simulink library "eop_grc"  (R2024a)
settings: Solver=VariableStepAuto  StartTime=0.0  StopTime=10.0  RelTol=1e-3
undefined symbols (not defined in the file or in its folder): AEOP_nReqMotSpdMax_X_A, AEOP_nRrOilTempSpdMod_X_degC, AEOP_nRrOilTempSpdMod_Y_KW, AEOP_nRrTMTempSpdMod_X_degC, EopC_bMotEnaMan_C, EopC_bMotEnaManTrig_C, EopC_nReqMotSpdMan_C, EopC_nReqMotSpdMin_C, EopC_nReqMotSpdTrig_C, EopC_rSpdRampDown_C, EopC_rSpdRampUp_C, EopC_volfDmd_A, MEOP_nReqMotSpdMax_Y_T, MEOP_nRrOilTempDetOptMod_Y_T, MEOP_nRrOilTempDetOptMod_Z_M, MEOP_nRrOilTempMotOptMod_Z_M, MEOP_nRrOilTempSpdMod_Z_M, MEOP_nRrTMTempMotOptMod_Y_T, MEOP_nRrTMTempSpdMod_Y_T
libraries: simulink x2
settings Model: Creator=FVT22063  LastModifiedBy=FVT22063

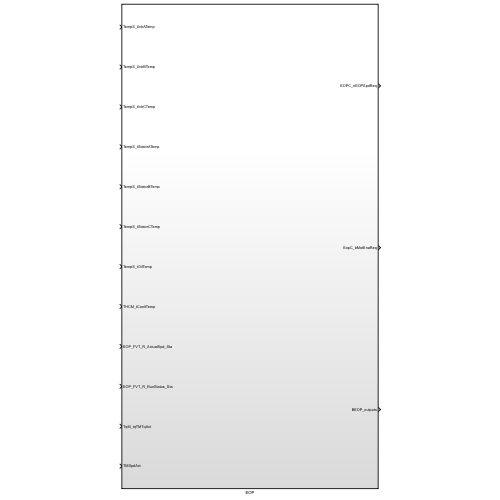
[thumbnail: Simulink's stored preview of the top-level diagram]
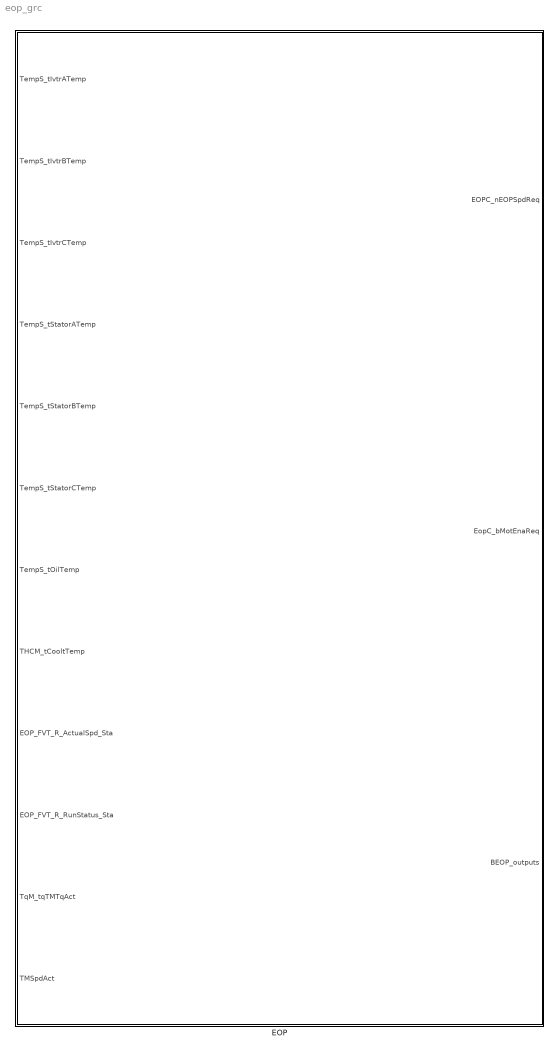
== system eop_grc ==
  EOP : Subsystem  TreatAsAtomicUnit=on
      settings: RTWSystemCode=Nonreusable function  RTWFcnNameOpts=Use subsystem name  RTWFileNameOpts=Use subsystem name

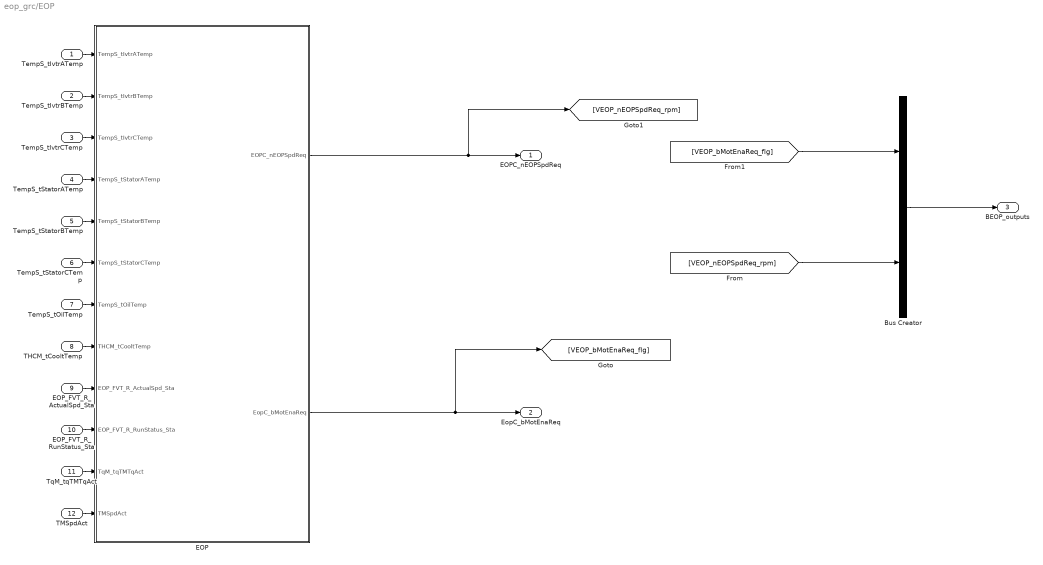
== system eop_grc/EOP ==
  TempS_tIvtrATemp : Inport
  TempS_tIvtrBTemp : Inport  Port=2
  TempS_tIvtrCTemp : Inport  Port=3
  TempS_tStatorATemp : Inport  Port=4
  TempS_tStatorBTemp : Inport  Port=5
  TempS_tStatorCTemp : Inport  Port=6
  TempS_tOilTemp : Inport  Port=7
  THCM_tCooltTemp : Inport  Port=8
  EOP_FVT_R_ActualSpd_Sta : Inport  Port=9
  EOP_FVT_R_RunStatus_Sta : Inport  Port=10
  TqM_tqTMTqAct : Inport  Port=11
  TMSpdAct : Inport  Port=12
  Bus Creator : BusCreator  Inputs=2  OutDataTypeStr=Bus: BEOP_outputs  NonVirtualBus=on
  EOP : Subsystem  TreatAsAtomicUnit=on
  EOPC_nEOPSpdReq : Outport
  EopC_bMotEnaReq : Outport  Port=2
  BEOP_outputs : Outport  Port=3  OutDataTypeStr=Bus: BEOP_outputs
  wires:
  TempS_tStatorBTemp/1 -> EOP/5(TempS_tStatorBTemp)
  TMSpdAct/1 -> EOP/12(TMSpdAct)
  EOP/2(EopC_bMotEnaReq) -> [VEOP_bMotEnaReq_flg], EopC_bMotEnaReq/1
  TempS_tStatorATemp/1 -> EOP/4(TempS_tStatorATemp)
  EOP_FVT_R_RunStatus_Sta/1 -> EOP/10(EOP_FVT_R_RunStatus_Sta)
  EOP_FVT_R_ActualSpd_Sta/1 -> EOP/9(EOP_FVT_R_ActualSpd_Sta)
  TqM_tqTMTqAct/1 -> EOP/11(TqM_tqTMTqAct)
  EOP/1(EOPC_nEOPSpdReq) -> [VEOP_nEOPSpdReq_rpm], EOPC_nEOPSpdReq/1
  TempS_tIvtrBTemp/1 -> EOP/2(TempS_tIvtrBTemp)
  THCM_tCooltTemp/1 -> EOP/8(THCM_tCooltTemp)
  TempS_tIvtrATemp/1 -> EOP/1(TempS_tIvtrATemp)
  TempS_tStatorCTemp/1 -> EOP/6(TempS_tStatorCTemp)
  TempS_tIvtrCTemp/1 -> EOP/3(TempS_tIvtrCTemp)
  TempS_tOilTemp/1 -> EOP/7(TempS_tOilTemp)
  Bus Creator/1 -> BEOP_outputs/1
  [VEOP_bMotEnaReq_flg] -> Bus Creator/1
  [VEOP_nEOPSpdReq_rpm] -> Bus Creator/2

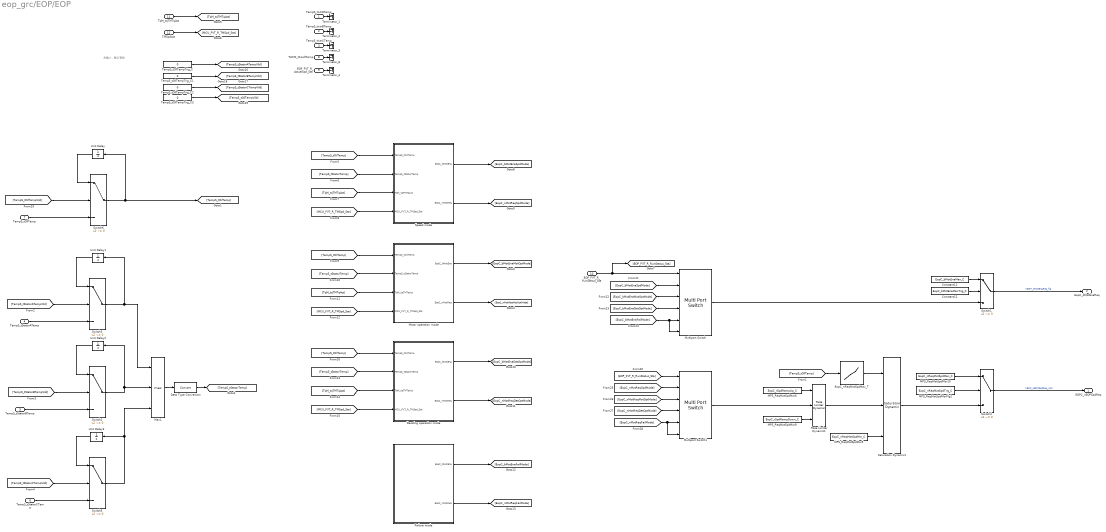
== system eop_grc/EOP/EOP ==
  note: 未输入，默认有效
  TempS_tIvtrATemp : Inport
  TempS_tIvtrBTemp : Inport  Port=2
  TempS_tIvtrCTemp : Inport  Port=3
  TempS_tStatorATemp : Inport  Port=4
  TempS_tStatorBTemp : Inport  Port=5
  TempS_tStatorCTemp : Inport  Port=6
  TempS_tOilTemp : Inport  Port=7
  THCM_tCooltTemp : Inport  Port=8
  EOP_FVT_R_ActualSpd_Sta : Inport  Port=9
  EOP_FVT_R_RunStatus_Sta : Inport  Port=10
  TqM_tqTMTqAct : Inport  Port=11
  TMSpdAct : Inport  Port=12
  Constant11 : Constant  Value=EopC_bMotEnaMan_C
  Constant12 : Constant  Value=EopC_bMotEnaManTrig_C
  Data Type Conversion : DataTypeConversion  SaturateOnIntegerOverflow=off  RndMeth=Floor
  Derating operation mode : Subsystem
  EopC_nReqMotSpdMax_T : Lookup_n-D  NumberOfTableDimensions=1  BreakpointsForDimension1=AEOP_nReqMotSpdMax_X_A  BreakpointsForDimension2=EopC_volfDmd_A  Table=MEOP_nReqMotSpdMax_Y_T  ExtrapMethod=Clip  UseLastTableValue=on  InternalRulePriority=Speed  RndMeth=Simplest
  Failure mode : Subsystem
  MPS_ReqMotSpdMor10 : Constant  Value=EopC_nReqMotSpdMan_C
  MPS_ReqMotSpdMor5 : Constant  Value=EopC_nReqMotSpdMin_C
  MPS_ReqMotSpdMor6 : Constant  Value=EopC_rSpdRampUp_C
  MPS_ReqMotSpdMor9 : Constant  Value=EopC_rSpdRampDown_C
  MPS_ReqMotSpdMorFlg1 : Constant  Value=EopC_nReqMotSpdTrig_C
  Max1 : MinMax  Function=max  Inputs=3
  Motor operation mode : Subsystem
  Multiport Switch : MultiPortSwitch  DataPortOrder=Specify indices  DataPortIndices={0,1,2,3}  DataPortForDefault=Additional data port  DiagnosticForDefault=None  SaturateOnIntegerOverflow=off  InputSameDT=off
  Multiport Switch1 : MultiPortSwitch  DataPortOrder=Zero-based contiguous  Inputs=4  DataPortIndices={EopStsCool.SpdMod, EopStsCool.MotOptMod,EopStsCool.DetOptMod,EopStsCool.FalMod}  DataPortForDefault=Additional data port  DiagnosticForDefault=None  zeroidx=on  SaturateOnIntegerOverflow=off  InputSameDT=off
  Rate Limiter Dynamic1 : simulink/Discontinuities/Rate Limiter Dynamic
  Saturation Dynamic1 : simulink/Discontinuities/Saturation Dynamic  OutMin=[]  OutMax=[]  OutDataTypeStr=Inherit: Same as second input  OutDataType=fixdt(1, 16)  OutScaling=2^-10  DoSatur=off
  Speed mode : Subsystem
  Switch{1..6} (6 alike) : Switch  Criteria=u2 ~= 0  SaturateOnIntegerOverflow=off  InputSameDT=off
  TempS_tOilTempTrig_C{,1..3} (4 alike) : Constant  Value=0
  Terminator_{1..4,8} (5 alike) : Terminator
  Unit Delay{,1..3} (4 alike) : UnitDelay  SampleTime=-1  HasFrameUpgradeWarning=on
  EOPC_nEOPSpdReq : Outport  VectorParamsAs1DForOutWhenUnconnected=off
  EopC_bMotEnaReq : Outport  Port=2  VectorParamsAs1DForOutWhenUnconnected=off
  wires:
  TempS_tIvtrATemp/1 -> Terminator_1/1
  TempS_tIvtrBTemp/1 -> Terminator_2/1
  TempS_tIvtrCTemp/1 -> Terminator_3/1
  TempS_tStatorATemp/1 -> Switch3/3
  THCM_tCooltTemp/1 -> Terminator_8/1
  Switch4/1 -> EOPC_nEOPSpdReq/1  "VEOP_nEOPSpdReq_rpm"
  MPS_ReqMotSpdMor9/1 -> Rate Limiter Dynamic1/3
  Speed mode/2(EopC_nMotReq) -> [EopC_nMotReqSpdMode]
  [EopC_nMotReqDetOptMode] -> Multiport Switch1/4
  [EopC_nMotReqSpdMode] -> Multiport Switch1/2
  [TempS_tOilTemp] -> EopC_nReqMotSpdMax_T/1
  [EopC_bMotEnaMotOptMode] -> Multiport Switch/3
  Speed mode/1(EopC_bMotEna) -> [EopC_bMotEnaSpdMode]
  [EopC_bMotEnaSpdMode] -> Multiport Switch/2
  EOP_FVT_R_RunStatus_Sta/1 -> Multiport Switch/1, [EOP_FVT_R_RunStatus_Sta]
  [EopC_nMotReqFailMode] -> Multiport Switch1/6, Multiport Switch1/5
  MPS_ReqMotSpdMorFlg1/1 -> Switch4/2
  Multiport Switch1/1 -> Rate Limiter Dynamic1/2
  TMSpdAct/1 -> [MCU_FVT_R_TMSpd_Sta]
  Constant12/1 -> Switch1/2
  MPS_ReqMotSpdMor5/1 -> Saturation Dynamic1/3
  [EopC_bMotEnaFailMode] -> Multiport Switch/6, Multiport Switch/5
  Saturation Dynamic1/1 -> Switch4/3
  [EopC_bMotEnaDetOptMode] -> Multiport Switch/4
  EopC_nReqMotSpdMax_T/1 -> Saturation Dynamic1/1
  Multiport Switch/1 -> Switch1/3
  Constant11/1 -> Switch1/1
  [EOP_FVT_R_RunStatus_Sta] -> Multiport Switch1/1
  Switch1/1 -> EopC_bMotEnaReq/1  "VEOP_bMotEnaReq_flg"
  MPS_ReqMotSpdMor10/1 -> Switch4/1
  MPS_ReqMotSpdMor6/1 -> Rate Limiter Dynamic1/1
  [EopC_nMotReqMotOptMode] -> Multiport Switch1/3
  TqM_tqTMTqAct/1 -> [TqM_tqTMTqAct]
  Rate Limiter Dynamic1/1 -> Saturation Dynamic1/2
  TempS_tOilTempTrig_C/1 -> [TempS_tStatorATempVild]
  TempS_tOilTempTrig_C1/1 -> [TempS_tStatorBTempVild]
  TempS_tOilTempTrig_C2/1 -> [TempS_tStatorCTempVild]
  TempS_tOilTempTrig_C3/1 -> [TempS_tOilTempVild]
  Switch3/1 -> Max1/1, Unit Delay1/1
  Unit Delay1/1 -> Switch3/1
  [TempS_tStatorATempVild] -> Switch3/2
  Unit Delay2/1 -> Switch2/1
  Switch2/1 -> Unit Delay2/1, Max1/2
  [TempS_tStatorBTempVild] -> Switch2/2
  TempS_tStatorBTemp/1 -> Switch2/3
  Switch5/1 -> Max1/3, Unit Delay3/1
  Unit Delay3/1 -> Switch5/1
  [TempS_tStatorCTempVild] -> Switch5/2
  TempS_tStatorCTemp/1 -> Switch5/3
  Unit Delay/1 -> Switch6/1
  Switch6/1 -> Unit Delay/1, [TempS_tOilTemp]
  [TempS_tOilTempVild] -> Switch6/2
  TempS_tOilTemp/1 -> Switch6/3
  [TempS_tOilTemp] -> Speed mode/1(TempS_tOilTemp)
  [TempS_tStatorTemp] -> Speed mode/2(TempS_tStatorTemp)
  [MCU_FVT_R_TMSpd_Sta] -> Speed mode/4(MCU_FVT_R_TMSpd_Sta)
  [TqM_tqTMTqAct] -> Speed mode/3(TqM_tqTMTqAct)
  [TqM_tqTMTqAct] -> Motor operation mode/3(TqM_tqTMTqAct)
  [MCU_FVT_R_TMSpd_Sta] -> Motor operation mode/4(MCU_FVT_R_TMSpd_Sta)
  [TempS_tStatorTemp] -> Motor operation mode/2(TempS_tStatorTemp)
  [TempS_tOilTemp] -> Motor operation mode/1(TempS_tOilTemp)
  Motor operation mode/1(EopC_bMotEna) -> [EopC_bMotEnaMotOptMode]
  Motor operation mode/2(EopC_nMotReq) -> [EopC_nMotReqMotOptMode]
  Derating operation mode/2(EopC_nMotReq) -> [EopC_nMotReqDetOptMode]
  Derating operation mode/1(EopC_bMotEna) -> [EopC_bMotEnaDetOptMode]
  [TempS_tOilTemp] -> Derating operation mode/1(TempS_tOilTemp)
  [TempS_tStatorTemp] -> Derating operation mode/2(TempS_tStatorTemp)
  [MCU_FVT_R_TMSpd_Sta] -> Derating operation mode/4(MCU_FVT_R_TMSpd_Sta)
  [TqM_tqTMTqAct] -> Derating operation mode/3(TqM_tqTMTqAct)
  Failure mode/1(EopC_bMotEna) -> [EopC_bMotEnaFailMode]
  Failure mode/2(EopC_nMotReq) -> [EopC_nMotReqFailMode]
  EOP_FVT_R_ActualSpd_Sta/1 -> Terminator_4/1
  Max1/1 -> Data Type Conversion/1
  Data Type Conversion/1 -> [TempS_tStatorTemp]

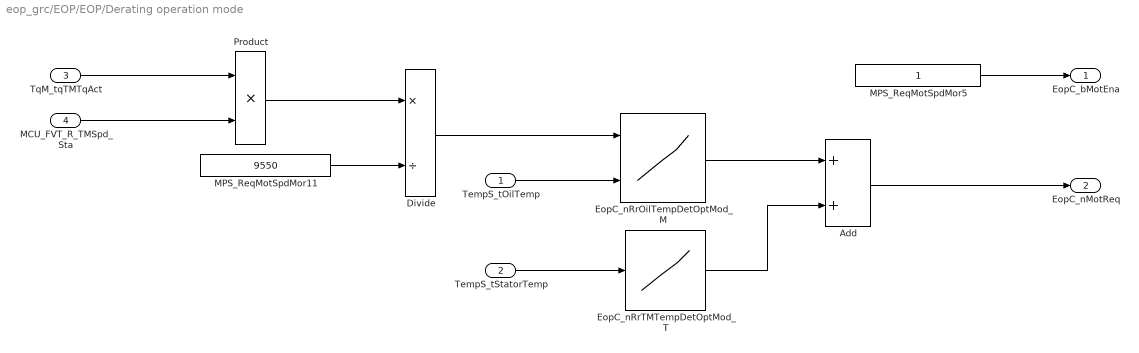
== system eop_grc/EOP/EOP/Derating operation mode ==
  TempS_tOilTemp : Inport
  TempS_tStatorTemp : Inport  Port=2
  TqM_tqTMTqAct : Inport  Port=3
  MCU_FVT_R_TMSpd_Sta : Inport  Port=4
  Add : Sum
  Divide : Product  Inputs=*/
  EopC_nRrOilTempDetOptMod_M : Lookup_n-D  BreakpointsForDimension1=AEOP_nRrOilTempSpdMod_Y_KW  BreakpointsForDimension2=AEOP_nRrOilTempSpdMod_X_degC  Table=MEOP_nRrOilTempDetOptMod_Z_M  ExtrapMethod=Clip  UseLastTableValue=on  InternalRulePriority=Speed  RndMeth=Simplest
      settings: InputPortMap=u0,u1
  EopC_nRrTMTempDetOptMod_T : Lookup_n-D  NumberOfTableDimensions=1  BreakpointsForDimension1=AEOP_nRrTMTempSpdMod_X_degC  BreakpointsForDimension2=EopC_volfDmd_A  Table=MEOP_nRrOilTempDetOptMod_Y_T  ExtrapMethod=Clip  UseLastTableValue=on  InternalRulePriority=Speed  RndMeth=Simplest
  MPS_ReqMotSpdMor11 : Constant  Value=9550  OutDataTypeStr=single
  MPS_ReqMotSpdMor5 : Constant  OutDataTypeStr=boolean
  Product : Product
  EopC_bMotEna : Outport  VectorParamsAs1DForOutWhenUnconnected=off
  EopC_nMotReq : Outport  Port=2  VectorParamsAs1DForOutWhenUnconnected=off
  wires:
  EopC_nRrTMTempDetOptMod_T/1 -> Add/2
  Divide/1 -> EopC_nRrOilTempDetOptMod_M/1
  EopC_nRrOilTempDetOptMod_M/1 -> Add/1
  MPS_ReqMotSpdMor5/1 -> EopC_bMotEna/1
  MPS_ReqMotSpdMor11/1 -> Divide/2
  Product/1 -> Divide/1
  Add/1 -> EopC_nMotReq/1
  TqM_tqTMTqAct/1 -> Product/1
  MCU_FVT_R_TMSpd_Sta/1 -> Product/2
  TempS_tStatorTemp/1 -> EopC_nRrTMTempDetOptMod_T/1
  TempS_tOilTemp/1 -> EopC_nRrOilTempDetOptMod_M/2

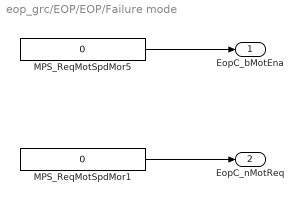
== system eop_grc/EOP/EOP/Failure mode ==
  MPS_ReqMotSpdMor1 : Constant  Value=0  OutDataTypeStr=single
  MPS_ReqMotSpdMor5 : Constant  Value=0  OutDataTypeStr=boolean
  EopC_bMotEna : Outport  VectorParamsAs1DForOutWhenUnconnected=off
  EopC_nMotReq : Outport  Port=2  VectorParamsAs1DForOutWhenUnconnected=off
  wires:
  MPS_ReqMotSpdMor1/1 -> EopC_nMotReq/1
  MPS_ReqMotSpdMor5/1 -> EopC_bMotEna/1

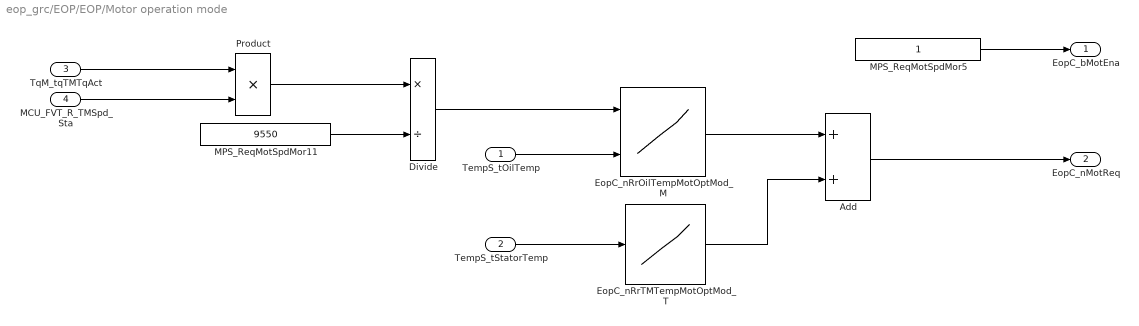
== system eop_grc/EOP/EOP/Motor operation mode ==
  TempS_tOilTemp : Inport
  TempS_tStatorTemp : Inport  Port=2
  TqM_tqTMTqAct : Inport  Port=3
  MCU_FVT_R_TMSpd_Sta : Inport  Port=4
  Add : Sum
  Divide : Product  Inputs=*/
  EopC_nRrOilTempMotOptMod_M : Lookup_n-D  BreakpointsForDimension1=AEOP_nRrOilTempSpdMod_Y_KW  BreakpointsForDimension2=AEOP_nRrOilTempSpdMod_X_degC  Table=MEOP_nRrOilTempMotOptMod_Z_M  ExtrapMethod=Clip  UseLastTableValue=on  InternalRulePriority=Speed  RndMeth=Simplest
      settings: InputPortMap=u0,u1
  EopC_nRrTMTempMotOptMod_T : Lookup_n-D  NumberOfTableDimensions=1  BreakpointsForDimension1=AEOP_nRrTMTempSpdMod_X_degC  BreakpointsForDimension2=EopC_volfDmd_A  Table=MEOP_nRrTMTempMotOptMod_Y_T  ExtrapMethod=Clip  UseLastTableValue=on  InternalRulePriority=Speed  RndMeth=Simplest
  MPS_ReqMotSpdMor11 : Constant  Value=9550  OutDataTypeStr=single
  MPS_ReqMotSpdMor5 : Constant  OutDataTypeStr=boolean
  Product : Product
  EopC_bMotEna : Outport  VectorParamsAs1DForOutWhenUnconnected=off
  EopC_nMotReq : Outport  Port=2  VectorParamsAs1DForOutWhenUnconnected=off
  wires:
  TempS_tOilTemp/1 -> EopC_nRrOilTempMotOptMod_M/2
  TempS_tStatorTemp/1 -> EopC_nRrTMTempMotOptMod_T/1
  MCU_FVT_R_TMSpd_Sta/1 -> Product/2
  TqM_tqTMTqAct/1 -> Product/1
  Add/1 -> EopC_nMotReq/1
  Product/1 -> Divide/1
  MPS_ReqMotSpdMor11/1 -> Divide/2
  MPS_ReqMotSpdMor5/1 -> EopC_bMotEna/1
  EopC_nRrOilTempMotOptMod_M/1 -> Add/1
  Divide/1 -> EopC_nRrOilTempMotOptMod_M/1
  EopC_nRrTMTempMotOptMod_T/1 -> Add/2

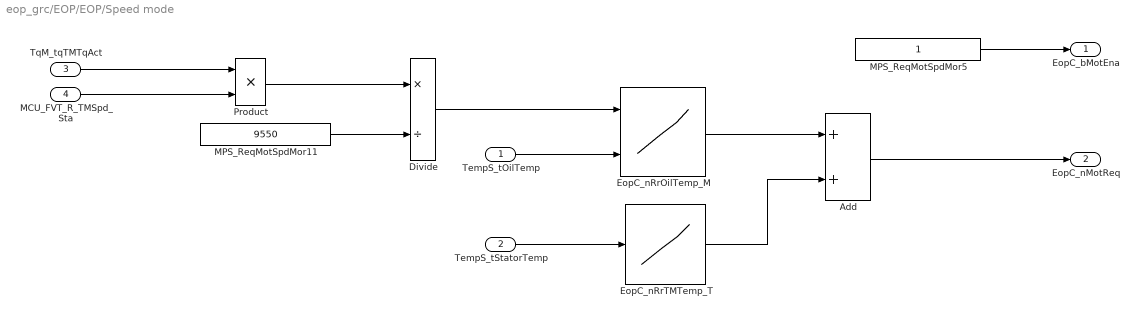
== system eop_grc/EOP/EOP/Speed mode ==
  TempS_tOilTemp : Inport
  TempS_tStatorTemp : Inport  Port=2
  TqM_tqTMTqAct : Inport  Port=3
  MCU_FVT_R_TMSpd_Sta : Inport  Port=4
  Add : Sum
  Divide : Product  Inputs=*/
  EopC_nRrOilTemp_M : Lookup_n-D  BreakpointsForDimension1=AEOP_nRrOilTempSpdMod_Y_KW  BreakpointsForDimension2=AEOP_nRrOilTempSpdMod_X_degC  Table=MEOP_nRrOilTempSpdMod_Z_M  ExtrapMethod=Clip  UseLastTableValue=on  InternalRulePriority=Speed  RndMeth=Simplest
      settings: InputPortMap=u0,u1
  EopC_nRrTMTemp_T : Lookup_n-D  NumberOfTableDimensions=1  BreakpointsForDimension1=AEOP_nRrTMTempSpdMod_X_degC  BreakpointsForDimension2=EopC_volfDmd_A  Table=MEOP_nRrTMTempSpdMod_Y_T  ExtrapMethod=Clip  UseLastTableValue=on  InternalRulePriority=Speed  RndMeth=Simplest
  MPS_ReqMotSpdMor11 : Constant  Value=9550  OutDataTypeStr=single
  MPS_ReqMotSpdMor5 : Constant  OutDataTypeStr=boolean
  Product : Product
  EopC_bMotEna : Outport  VectorParamsAs1DForOutWhenUnconnected=off
  EopC_nMotReq : Outport  Port=2  VectorParamsAs1DForOutWhenUnconnected=off
  wires:
  EopC_nRrTMTemp_T/1 -> Add/2
  Divide/1 -> EopC_nRrOilTemp_M/1
  EopC_nRrOilTemp_M/1 -> Add/1
  MPS_ReqMotSpdMor5/1 -> EopC_bMotEna/1
  MPS_ReqMotSpdMor11/1 -> Divide/2
  Product/1 -> Divide/1
  Add/1 -> EopC_nMotReq/1
  TqM_tqTMTqAct/1 -> Product/1
  MCU_FVT_R_TMSpd_Sta/1 -> Product/2
  TempS_tStatorTemp/1 -> EopC_nRrTMTemp_T/1
  TempS_tOilTemp/1 -> EopC_nRrOilTemp_M/2
